simulink model "tst_bus_simple_combined"  (Simulink 8.0)
settings: Solver=ode45  StartTime=0.0  StopTime=10.0  RelTol=1e-3
settings Model: Creator=Marci  LastModifiedBy=Marci

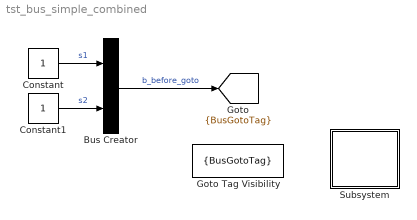
== system tst_bus_simple_combined ==
  Bus Creator : BusCreator  Inputs=2
  Constant : Constant
  Constant1 : Constant
  Goto Tag Visibility : GotoTagVisibility  GotoTag=BusGotoTag
  Subsystem : Subsystem
  tag scope: BusGotoTag=scoped
  wires:
  Constant1/1 -> Bus Creator/2  "s2"
  Constant/1 -> Bus Creator/1  "s1"
  Bus Creator/1 -> [BusGotoTag]  "b_before_goto"

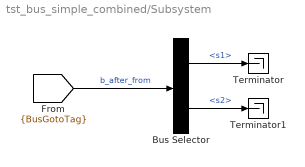
== system tst_bus_simple_combined/Subsystem ==
  Bus Selector : BusSelector  OutputSignals=s1,s2
  Terminator : Terminator
  Terminator1 : Terminator
  wires:
  Bus Selector/2 -> Terminator1/1  "<s2>"
  Bus Selector/1 -> Terminator/1  "<s1>"
  [BusGotoTag] -> Bus Selector/1  "b_after_from"
